simulink model "15c_fir_iir_realization"  (R2023b)
settings: Solver=VariableStepAuto  StartTime=0.0  StopTime=10.0  RelTol=1e-3
libraries: dspsrcs4 x1
settings Model: Creator=HP  LastModifiedBy=HP

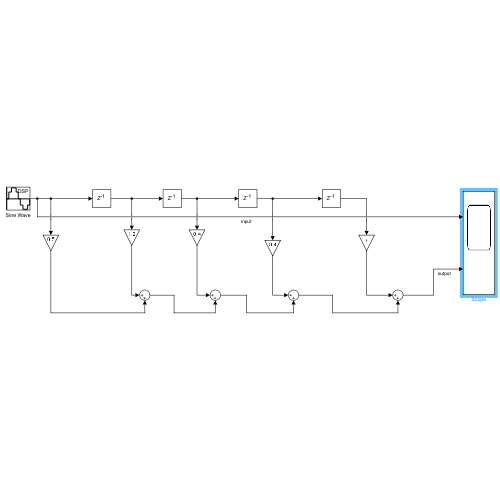
[thumbnail: Simulink's stored preview of the top-level diagram]
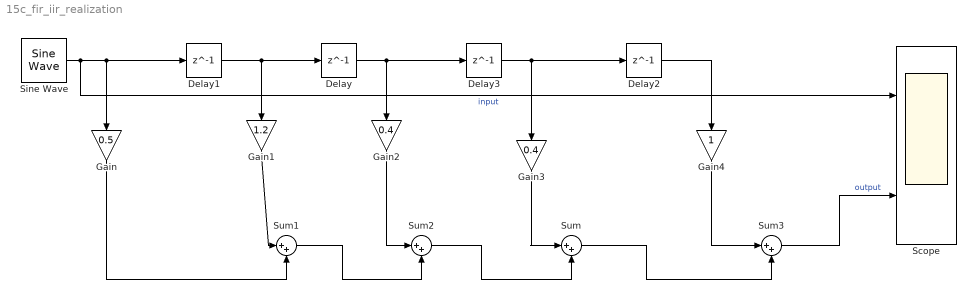
== system 15c_fir_iir_realization ==
  Delay{,1..3} (4 alike) : Delay  DelayLength=1  InitialCondition=0
  Gain : Gain  Gain=0.5
  Gain1 : Gain  Gain=1.2
  Gain2 : Gain  Gain=0.4
  Gain3 : Gain  Gain=0.4
  Gain4 : Gain
  Scope : Scope  NumInputPorts=2
  Sine Wave : dspsrcs4/Sine Wave  Amplitude=1  Frequency=100  Phase=0  SampleMode=Discrete  OutComplex=Real  CompMethod=Trigonometric fcn  TableSize=Speed  SampleTime=1/1000  SamplesPerFrame=1  ResetState=Restart at time zero  OutputFrames=off  dataType=double  wordLen=16  udDataType=sfix(16)  fracBitsMode=Best precision  numFracBits=15  OutDataTypeStr=double  LastOutDataTypeStr=double
  Sum{,1..3} (4 alike) : Sum  Inputs=|++
  wires:
  Sine Wave/1 -> Scope/1, Gain/1, Delay1/1  "input"
  Delay1/1 -> Gain1/1, Delay/1
  Delay/1 -> Delay3/1, Gain2/1
  Delay3/1 -> Gain3/1, Delay2/1
  Delay2/1 -> Gain4/1
  Sum1/1 -> Sum2/2
  Sum2/1 -> Sum/2
  Sum/1 -> Sum3/2
  Gain/1 -> Sum1/2
  Gain1/1 -> Sum1/1
  Gain2/1 -> Sum2/1
  Gain3/1 -> Sum/1
  Gain4/1 -> Sum3/1
  Sum3/1 -> Scope/2  "output"
